simulink model "Sim_PA_DDPG_4drone"  (R2025a)
settings: Solver=ode1  StartTime=0.0  StopTime=Tf  FixedStep=Ts_Sim  RelTol=1e-3
undefined symbols (not defined in the file): control_noise, p_IC, phi_IC, phi_limit, pqr_Limit, psi_dsr, psi_IC, psi_limit, q_IC, r_IC, saturation_logic, state_noise, theta_IC, theta_limit, Ts_Sim, u_IC, uvw_Limit, v_IC, w_IC, wind_logic, x_IC, xy_Limit, y_IC, z_IC, z_Limit
libraries: rllib x8
(part 2 of 2)

== matlab function Sim_PA_DDPG_4drone/leader 1/System Solver/System Solver ==
  data: roll output; pitch output; r_yaw output; ft output; u1 input; u2 input; u3 input; Ts input; r_yaw input
function [roll, pitch, r_yaw, ft ] = system_solver(u1, u2, u3, Ts, r_yaw)

    m = 1; g = 9.81;
    
    ft = m * sqrt( u1^2 + u2^2 + (u3-g)^2 );

    % a = sin(r_yaw);
    % b = cos(r_yaw);
    % 
    % A = u1 / (u3);
    % B = u2 / (u3);
    % C = (a*A - b*B) / ( (a^2) + (b^2)) ;
    % 
    % roll = atan( (B + b*C) / a );
    % pitch = atan( C * cos(roll) );

    roll = asin( (u2*m) / ft );
    pitch = asin( (-u1*m) / (ft*cos(roll)) );
    r_yaw = 0;

    % Smoothing Factor ( Use exponential decay, just to start from zero )
    % roll = roll * (1-exp(-Ts));
    % pitch = pitch * (1-exp(-Ts));
    % r_yaw = r_yaw * (1-exp(-Ts));

    % Saturation
    if roll > pi/10
        roll = pi/10;
    elseif roll < -pi/10
        roll = -pi/10;
    end

    if pitch > pi/10
        pitch = pi/10;
    elseif pitch < -pi/10
        pitch = -pi/10;
    end

end

% function [ft, pitch, roll] = system_solve(u1, u2, u3, psi, m) % u1 = ux , u2 = uy , u3 = uz - g  
%     if psi <= 0.001 && psi >= -0.001
%         psi = 0.001;
%     end
%     a = sin(psi);
%     b = cos(psi);
% 
%     A = u1 / (u3);
%     B = u2 / (u3);
%     C = (a*A - b*B) / ( (a^2) + (b^2)) ;
% 
%     roll = atan( (B + b*C) / a );
%     pitch = atan( C * cos(roll) );
% 
%     % saftey limit threshold on desired pitch and roll
%     if pitch>pi/4
%         pitch = pi/4;
%     elseif pitch<-pi/4
%         pitch = -pi/4;
%     end
%     if roll>pi/4
%         roll = pi/4;
%     elseif roll<-pi/4
%         roll = -pi/4;
%     end
%     ft = ( m / (cos(pitch)*cos(roll)) ) * (-u3); 
% end

== matlab function Sim_PA_DDPG_4drone/leader 1/Attitude DDPG/Attitude Error ==
  data: phi_dsr input; phi_dot_dsr input; theta_dsr input; theta_dot_dsr input; psi_dsr input; psi_dot_dsr input; phi input; theta input; psi input; e_phi output; e_theta output; e_psi output; phi_dot input; theta_dot input; psi_dot input; e_phi_dot output; e_theta_dot output; e_psi_dot output
function [ e_phi, e_theta, e_psi, e_phi_dot, e_theta_dot, e_psi_dot ] = calculate_errors(phi_dsr, phi_dot_dsr, theta_dsr, theta_dot_dsr, psi_dsr, psi_dot_dsr, phi, theta, psi, phi_dot, theta_dot, psi_dot)
   
    e_phi = phi_dsr - phi;
    e_theta = theta_dsr - theta;
    e_psi = psi_dsr - psi;

    e_phi_dot = phi_dot_dsr - phi_dot;
    e_theta_dot = theta_dot_dsr - theta_dot;
    e_psi_dot = psi_dot_dsr - psi_dot;

end

== matlab function Sim_PA_DDPG_4drone/leader 1/Position DDPG/Position Error ==
  data: x_desired input; y_desired input; z_desired input; xdot_desired input; ydot_desired input; zdot_desired input; x input; y input; z input; e_x output; e_y output; e_z output; xdot input; ydot input; zdot input; e_xdot output; e_ydot output; e_zdot output
function [e_x, e_y, e_z, e_xdot, e_ydot, e_zdot] = ...
      calculate_errors(x_desired, y_desired, z_desired, ...
      xdot_desired, ydot_desired, zdot_desired, ...
      x,y,z, xdot,ydot,zdot)

    e_x    = x_desired - x;
    e_y    = y_desired - y;
    e_z    = z_desired - z;
    e_xdot = xdot_desired - xdot;
    e_ydot = ydot_desired - ydot;
    e_zdot = zdot_desired - zdot;
    
end

% formal is Actual - Reference

== matlab function Sim_PA_DDPG_4drone/leader 1/Position DDPG/MATLAB Function ==
  data: e_x input; r output; e_y input; e_z input; e_u input; e_v input; e_w input; u_dot input; v_dot input; w_dot input; isdone output
function [r,isdone] = calculate_reward(e_x, e_y, e_z, e_u, e_v, e_w, u_dot, v_dot, w_dot)

    r = -    1*( abs(e_x)   + abs(e_y)   + abs(e_z) ) ...
        -  0.1*( abs(e_u)   + abs(e_v)   + abs(e_w) ) ...
        - 0.01*( abs(u_dot) + abs(v_dot) + abs(w_dot) );
    
   isdone = 0;
   
end

== matlab function Sim_PA_DDPG_4drone/leader 1/Attitude DDPG/MATLAB Function ==
  data: e_phi input; r output; e_theta input; e_psi input; e_phi_dot input; e_theta_dot input; e_psi_dot input; tau_x input; tau_y input; tau_z input; isdone output
function [r,isdone] = calculate_reward(e_phi, e_theta, e_psi, e_phi_dot, e_theta_dot, e_psi_dot, tau_x, tau_y, tau_z )

    Error_Angle      =    2*( abs(e_phi)     +  abs(e_theta)     + abs(e_psi) );
    Error_Angle_Rate =  0.1*( abs(e_phi_dot) +  abs(e_theta_dot) + abs(e_psi_dot) );
    Action           = 0.01*( abs(tau_x)     +  abs(tau_y)       + abs(tau_z) );

    r = - Error_Angle - Error_Angle_Rate - Action;

    isdone = (abs(e_phi) > 100) || (abs(e_theta) > 100) || (abs(e_psi) > 100);
end

== matlab function Sim_PA_DDPG_4drone/drone 2/Attitude DDPG/MATLAB Function ==
  data: e_phi input; r output; e_theta input; e_psi input; e_phi_dot input; e_theta_dot input; e_psi_dot input; tau_x input; tau_y input; tau_z input; isdone output
function [r,isdone] = calculate_reward(e_phi, e_theta, e_psi, e_phi_dot, e_theta_dot, e_psi_dot, tau_x, tau_y, tau_z )

    Error_Angle      =    2*( abs(e_phi)     +  abs(e_theta)     + abs(e_psi) );
    Error_Angle_Rate =  0.1*( abs(e_phi_dot) +  abs(e_theta_dot) + abs(e_psi_dot) );
    Action           = 0.01*( abs(tau_x)     +  abs(tau_y)       + abs(tau_z) );

    r = - Error_Angle - Error_Angle_Rate - Action;

    isdone = (abs(e_phi) > 100) || (abs(e_theta) > 100) || (abs(e_psi) > 100);
end

== matlab function Sim_PA_DDPG_4drone/drone 2/Drone Dynamics/MATLAB Function ==
  data: ft input; u_dot output; phi input; theta input; psi input; v_dot output; w_dot output
function [u_dot, v_dot, w_dot] = fcn(ft,phi,theta,psi)

m = 1; g = 9.81;

u_dot = -(ft/m)*( sin(phi)*sin(psi) + cos(phi)*cos(psi)*sin(theta) ); 
v_dot = -(ft/m)*( cos(phi)*sin(psi)*sin(theta) - cos(psi)*sin(phi));
w_dot = g-(ft/m)*( cos(phi)*cos(theta) );

end

== matlab function Sim_PA_DDPG_4drone/drone 2/Drone Dynamics/MATLAB Function1 ==
  data: tau_x input; p_dot output; tau_y input; tau_z input; p input; q_dot output; r_dot output; q input; r input
function [p_dot, q_dot, r_dot] = fcn(tau_x,tau_y,tau_z,p,q,r)

Ix = 0.3; Iy = 0.4; Iz = 0.5; 

p_dot = ((Iy-Iz)*q*r/Ix)  + tau_x/Ix;
q_dot = ((Iz-Ix)*p*r/Iy)  + tau_y/Iy;
r_dot = ((Ix-Iy)*p*q/Iz)  + tau_z/Iz;


end

== matlab function Sim_PA_DDPG_4drone/drone 2/Drone Dynamics/MATLAB Function2 ==
  data: p input; q input; r input; phi_dot output; phi input; theta input; theta_dot output; psi_dot output
function [phi_dot, theta_dot, psi_dot] = fcn(p,q,r, phi,theta)

    phi_dot   = p + (q*sin(phi)*tan(theta)) + (r*cos(phi)*tan(theta));
    theta_dot = (q*cos(phi)) - (r*sin(phi));
    psi_dot   = (q*sin(phi)/cos(theta)) + (r*cos(phi)/cos(theta));

end



    % if theta == deg2rad(90) || theta == deg2rad(-90)
    %    theta = sign(theta)*deg2rad(89.9); 
    % end

% 89.9 value is fixed. 
% if change to 89.99, phi_dot and psi_dot value will explode.

== matlab function Sim_PA_DDPG_4drone/drone 2/Drone Dynamics/MATLAB Function3 ==
  settings: updateMethod=DISCRETE
  data: state_vector input; noisy_vector output; noise_percent input
function noisy_vector = add_state_noise(state_vector,noise_percent)

    sensor_uncert = [0.02, 0.02, 0.05, 0.05, 0.05, 0.05, 0.15, 0.15, 0.5, 0.005, 0.005, 0.005]';
  
    noise = (noise_percent) * sensor_uncert .* randn(size(state_vector)); % 0.01 usually add noise_percent 1 2 3 4 5
    noisy_vector = state_vector + noise;

end

== matlab function Sim_PA_DDPG_4drone/drone 2/Drone Dynamics/MATLAB Function4 ==
  settings: updateMethod=DISCRETE
  data: control_vector input; noisy_vector output; noise_percent input
function noisy_vector = add_control_noise(control_vector, noise_percent)

    L = 0.2;
    % drag = 0.02; % (drag coef)
    max_Ft = 2*9.81;
    Tmax = max_Ft/4;
    Max_torque = Tmax*L*2;
    actuator_uncert = [0.1*max_Ft, 0.01*Max_torque, 0.01*Max_torque, 0.02*Max_torque]';
    
    noise = (noise_percent) * actuator_uncert .* randn(size(control_vector)); % noise_percent 1 2 3 4 5
    noisy_vector = control_vector + noise;
    
end

== matlab function Sim_PA_DDPG_4drone/drone 2/Drone Dynamics/MATLAB Function5 ==
  data: X input; Wxyz input; X output; Ts_Sim input; wind_logic input
function X = wind_f_m( X,Wxyz, Ts_Sim,  wind_logic)

    Cd = [.8; 0.8;1.2]; % Drag coefficient
    L = 0.2; % Half arm length (m)
    h = 0.05;
    A = [L*2*h, L*2*h, 2*L*L]; % Approximate frontal areas [x, y, z] in m^2
    r = [ L,  L, -L, -L;   % X positions of motors
          L, -L, -L,  L;   % Y positions of motors
          0,  0,  0,  0 ]; % Z positions (motors at same height)
    rho = 1.225; % Air density (kg/m^3)

    Ix = 0.3; Iy = 0.4; Iz = 0.5; m = 1;
    if wind_logic ==1
        R = eul2rotm_zyx( X(7), X(8), X(9) );
        Wxyz_body = R'*Wxyz;
        V_rel = X(4:6) - Wxyz_body;
        F_wind = -0.5 * rho * Cd .*diag(A) * (V_rel .* abs(V_rel)); % Compute wind forces
        
        F_wind_motors = repmat(F_wind, 1, 4) + 0.01*randn(3,4);
    
        M_wind_motors = cross(r, F_wind_motors, 1);
        M_wind = sum(M_wind_motors, 2);  
        
        accn_dist = F_wind/m;
        alpha_dist=    [M_wind(1)/Ix;
                        M_wind(2)/Iy;
                        M_wind(3)/Iz];
    
        X = X + Ts_Sim * [0;0;0;
                         accn_dist;
                         0;0;0;
                         alpha_dist];
    end
end

== matlab function Sim_PA_DDPG_4drone/drone 2/Drone Dynamics/MATLAB Function6 ==
  data: U input; out output; logic input
% saturation function
function out = saturate_controls(U, logic)

    if logic == 1

        ft = U(1);
        torques = [U(2); U(3); U(4)];
        m = 1;
        g = 9.81;
        L = 0.2;
        drag = 0.02; % (drag coef)
        max_Ft = 2*m*g;
        Tmin = 0;
        Tmax = max_Ft/4;
        max_torque = Tmax*L*2;
        max_yaw_torque = 0.7*max_torque;

        % saturate the torques to the max torque the drone can produce
        for p = 1:2 % sat the first 2
            if torques(p) > max_torque
                torques(p) = max_torque;
            elseif torques(p) < -max_torque
                torques(p) = -max_torque;
            end
        end
        if torques(3) > max_yaw_torque
            torques(3) = max_yaw_torque;
        elseif torques(3) < -max_yaw_torque
            torques(3) = -max_yaw_torque;
        end
        % solve for the thrust of each motor given those torques
        T1 = (ft - torques(1)/(2*L) - torques(2)/(2*L) + torques(3)/(4*drag)) / 4;
        T2 = (ft - torques(1)/(2*L) + torques(2)/(2*L) + torques(3)/(4*drag)) / 4;
        T3 = (ft + torques(1)/(2*L) - torques(2)/(2*L) - torques(3)/(4*drag)) / 4;
        T4 = (ft + torques(1)/(2*L) + torques(2)/(2*L) - torques(3)/(4*drag)) / 4;
        each_motor_thrust = [T1;T2;T3;T4];

        % saturate each motor thrust to its bounded values
        for j = 1:4
            if each_motor_thrust(j) > Tmax
                each_motor_thrust(j) = Tmax;
            elseif each_motor_thrust(j) < Tmin
                each_motor_thrust(j) = Tmin;
            end
        end

        ft = sum(each_motor_thrust);

        if ft>max_Ft
            ft = max_Ft;
        elseif ft<0
            ft = 0;
        end

        out = [ft; torques];

    else
    
        out = U;
    
    end


end

== matlab function Sim_PA_DDPG_4drone/drone 2/Position DDPG/MATLAB Function ==
  data: e_x input; r output; e_y input; e_z input; e_u input; e_v input; e_w input; u_dot input; v_dot input; w_dot input; isdone output
function [r,isdone] = calculate_reward(e_x, e_y, e_z, e_u, e_v, e_w, u_dot, v_dot, w_dot)

    r = -    1*( abs(e_x)   + abs(e_y)   + abs(e_z) ) ...
        -  0.1*( abs(e_u)   + abs(e_v)   + abs(e_w) ) ...
        - 0.01*( abs(u_dot) + abs(v_dot) + abs(w_dot) );
    
   isdone = 0;
   
end

== matlab function Sim_PA_DDPG_4drone/leader 1/Drone Dynamics/MATLAB Function1 ==
  data: tau_x input; p_dot output; tau_y input; tau_z input; p input; q_dot output; r_dot output; q input; r input
function [p_dot, q_dot, r_dot] = fcn(tau_x,tau_y,tau_z,p,q,r)

Ix = 0.3; Iy = 0.4; Iz = 0.5; 

p_dot = ((Iy-Iz)*q*r/Ix)  + tau_x/Ix;
q_dot = ((Iz-Ix)*p*r/Iy)  + tau_y/Iy;
r_dot = ((Ix-Iy)*p*q/Iz)  + tau_z/Iz;


end

== matlab function Sim_PA_DDPG_4drone/drone 2/Position DDPG/Position Error ==
  data: x_desired input; y_desired input; z_desired input; xdot_desired input; ydot_desired input; zdot_desired input; x input; y input; z input; e_x output; e_y output; e_z output; xdot input; ydot input; zdot input; e_xdot output; e_ydot output; e_zdot output
function [e_x, e_y, e_z, e_xdot, e_ydot, e_zdot] = ...
      calculate_errors(x_desired, y_desired, z_desired, ...
      xdot_desired, ydot_desired, zdot_desired, ...
      x,y,z, xdot,ydot,zdot)

    e_x    = x_desired - x;
    e_y    = y_desired - y;
    e_z    = z_desired - z;
    e_xdot = xdot_desired - xdot;
    e_ydot = ydot_desired - ydot;
    e_zdot = zdot_desired - zdot;
    
end

% formal is Actual - Reference

== matlab function Sim_PA_DDPG_4drone/drone 2/System Solver/System Solver ==
  data: roll output; pitch output; r_yaw output; ft output; u1 input; u2 input; u3 input; Ts input; r_yaw input
function [roll, pitch, r_yaw, ft ] = system_solver(u1, u2, u3, Ts, r_yaw)

    m = 1; g = 9.81;
    
    ft = m * sqrt( u1^2 + u2^2 + (u3-g)^2 );

    % a = sin(r_yaw);
    % b = cos(r_yaw);
    % 
    % A = u1 / (u3);
    % B = u2 / (u3);
    % C = (a*A - b*B) / ( (a^2) + (b^2)) ;
    % 
    % roll = atan( (B + b*C) / a );
    % pitch = atan( C * cos(roll) );

    roll = asin( (u2*m) / ft );
    pitch = asin( (-u1*m) / (ft*cos(roll)) );
    r_yaw = 0;

    % Smoothing Factor ( Use exponential decay, just to start from zero )
    % roll = roll * (1-exp(-Ts));
    % pitch = pitch * (1-exp(-Ts));
    % r_yaw = r_yaw * (1-exp(-Ts));

    % Saturation
    if roll > pi/10
        roll = pi/10;
    elseif roll < -pi/10
        roll = -pi/10;
    end

    if pitch > pi/10
        pitch = pi/10;
    elseif pitch < -pi/10
        pitch = -pi/10;
    end

end

% function [ft, pitch, roll] = system_solve(u1, u2, u3, psi, m) % u1 = ux , u2 = uy , u3 = uz - g  
%     if psi <= 0.001 && psi >= -0.001
%         psi = 0.001;
%     end
%     a = sin(psi);
%     b = cos(psi);
% 
%     A = u1 / (u3);
%     B = u2 / (u3);
%     C = (a*A - b*B) / ( (a^2) + (b^2)) ;
% 
%     roll = atan( (B + b*C) / a );
%     pitch = atan( C * cos(roll) );
% 
%     % saftey limit threshold on desired pitch and roll
%     if pitch>pi/4
%         pitch = pi/4;
%     elseif pitch<-pi/4
%         pitch = -pi/4;
%     end
%     if roll>pi/4
%         roll = pi/4;
%     elseif roll<-pi/4
%         roll = -pi/4;
%     end
%     ft = ( m / (cos(pitch)*cos(roll)) ) * (-u3); 
% end

== matlab function Sim_PA_DDPG_4drone/drone 3/Attitude DDPG/Attitude Error ==
  data: phi_dsr input; phi_dot_dsr input; theta_dsr input; theta_dot_dsr input; psi_dsr input; psi_dot_dsr input; phi input; theta input; psi input; e_phi output; e_theta output; e_psi output; phi_dot input; theta_dot input; psi_dot input; e_phi_dot output; e_theta_dot output; e_psi_dot output
function [ e_phi, e_theta, e_psi, e_phi_dot, e_theta_dot, e_psi_dot ] = calculate_errors(phi_dsr, phi_dot_dsr, theta_dsr, theta_dot_dsr, psi_dsr, psi_dot_dsr, phi, theta, psi, phi_dot, theta_dot, psi_dot)
   
    e_phi = phi_dsr - phi;
    e_theta = theta_dsr - theta;
    e_psi = psi_dsr - psi;

    e_phi_dot = phi_dot_dsr - phi_dot;
    e_theta_dot = theta_dot_dsr - theta_dot;
    e_psi_dot = psi_dot_dsr - psi_dot;

end

== matlab function Sim_PA_DDPG_4drone/drone 3/Attitude DDPG/MATLAB Function ==
  data: e_phi input; r output; e_theta input; e_psi input; e_phi_dot input; e_theta_dot input; e_psi_dot input; tau_x input; tau_y input; tau_z input; isdone output
function [r,isdone] = calculate_reward(e_phi, e_theta, e_psi, e_phi_dot, e_theta_dot, e_psi_dot, tau_x, tau_y, tau_z )

    Error_Angle      =    2*( abs(e_phi)     +  abs(e_theta)     + abs(e_psi) );
    Error_Angle_Rate =  0.1*( abs(e_phi_dot) +  abs(e_theta_dot) + abs(e_psi_dot) );
    Action           = 0.01*( abs(tau_x)     +  abs(tau_y)       + abs(tau_z) );

    r = - Error_Angle - Error_Angle_Rate - Action;

    isdone = (abs(e_phi) > 100) || (abs(e_theta) > 100) || (abs(e_psi) > 100);
end

== matlab function Sim_PA_DDPG_4drone/drone 3/Drone Dynamics/MATLAB Function ==
  data: ft input; u_dot output; phi input; theta input; psi input; v_dot output; w_dot output
function [u_dot, v_dot, w_dot] = fcn(ft,phi,theta,psi)

m = 1; g = 9.81;

u_dot = -(ft/m)*( sin(phi)*sin(psi) + cos(phi)*cos(psi)*sin(theta) ); 
v_dot = -(ft/m)*( cos(phi)*sin(psi)*sin(theta) - cos(psi)*sin(phi));
w_dot = g-(ft/m)*( cos(phi)*cos(theta) );

end

== matlab function Sim_PA_DDPG_4drone/drone 3/Drone Dynamics/MATLAB Function1 ==
  data: tau_x input; p_dot output; tau_y input; tau_z input; p input; q_dot output; r_dot output; q input; r input
function [p_dot, q_dot, r_dot] = fcn(tau_x,tau_y,tau_z,p,q,r)

Ix = 0.3; Iy = 0.4; Iz = 0.5; 

p_dot = ((Iy-Iz)*q*r/Ix)  + tau_x/Ix;
q_dot = ((Iz-Ix)*p*r/Iy)  + tau_y/Iy;
r_dot = ((Ix-Iy)*p*q/Iz)  + tau_z/Iz;


end

== matlab function Sim_PA_DDPG_4drone/drone 3/Drone Dynamics/MATLAB Function2 ==
  data: p input; q input; r input; phi_dot output; phi input; theta input; theta_dot output; psi_dot output
function [phi_dot, theta_dot, psi_dot] = fcn(p,q,r, phi,theta)

    phi_dot   = p + (q*sin(phi)*tan(theta)) + (r*cos(phi)*tan(theta));
    theta_dot = (q*cos(phi)) - (r*sin(phi));
    psi_dot   = (q*sin(phi)/cos(theta)) + (r*cos(phi)/cos(theta));

end



    % if theta == deg2rad(90) || theta == deg2rad(-90)
    %    theta = sign(theta)*deg2rad(89.9); 
    % end

% 89.9 value is fixed. 
% if change to 89.99, phi_dot and psi_dot value will explode.

== matlab function Sim_PA_DDPG_4drone/drone 3/Drone Dynamics/MATLAB Function3 ==
  settings: updateMethod=DISCRETE
  data: state_vector input; noisy_vector output; noise_percent input
function noisy_vector = add_state_noise(state_vector,noise_percent)

    sensor_uncert = [0.02, 0.02, 0.05, 0.05, 0.05, 0.05, 0.15, 0.15, 0.5, 0.005, 0.005, 0.005]';
  
    noise = (noise_percent) * sensor_uncert .* randn(size(state_vector)); % 0.01 usually add noise_percent 1 2 3 4 5
    noisy_vector = state_vector + noise;

end

== matlab function Sim_PA_DDPG_4drone/drone 3/Drone Dynamics/MATLAB Function4 ==
  settings: updateMethod=DISCRETE
  data: control_vector input; noisy_vector output; noise_percent input
function noisy_vector = add_control_noise(control_vector, noise_percent)

    L = 0.2;
    % drag = 0.02; % (drag coef)
    max_Ft = 2*9.81;
    Tmax = max_Ft/4;
    Max_torque = Tmax*L*2;
    actuator_uncert = [0.1*max_Ft, 0.01*Max_torque, 0.01*Max_torque, 0.02*Max_torque]';
    
    noise = (noise_percent) * actuator_uncert .* randn(size(control_vector)); % noise_percent 1 2 3 4 5
    noisy_vector = control_vector + noise;
    
end

== matlab function Sim_PA_DDPG_4drone/leader 1/Drone Dynamics/MATLAB Function ==
  data: ft input; u_dot output; phi input; theta input; psi input; v_dot output; w_dot output
function [u_dot, v_dot, w_dot] = fcn(ft,phi,theta,psi)

m = 1; g = 9.81;

u_dot = -(ft/m)*( sin(phi)*sin(psi) + cos(phi)*cos(psi)*sin(theta) ); 
v_dot = -(ft/m)*( cos(phi)*sin(psi)*sin(theta) - cos(psi)*sin(phi));
w_dot = g-(ft/m)*( cos(phi)*cos(theta) );

end

== matlab function Sim_PA_DDPG_4drone/drone 3/Drone Dynamics/MATLAB Function5 ==
  data: X input; Wxyz input; X output; Ts_Sim input; wind_logic input
function X = wind_f_m( X,Wxyz, Ts_Sim,  wind_logic)

    Cd = [.8; 0.8;1.2]; % Drag coefficient
    L = 0.2; % Half arm length (m)
    h = 0.05;
    A = [L*2*h, L*2*h, 2*L*L]; % Approximate frontal areas [x, y, z] in m^2
    r = [ L,  L, -L, -L;   % X positions of motors
          L, -L, -L,  L;   % Y positions of motors
          0,  0,  0,  0 ]; % Z positions (motors at same height)
    rho = 1.225; % Air density (kg/m^3)

    Ix = 0.3; Iy = 0.4; Iz = 0.5; m = 1;
    if wind_logic ==1
        R = eul2rotm_zyx( X(7), X(8), X(9) );
        Wxyz_body = R'*Wxyz;
        V_rel = X(4:6) - Wxyz_body;
        F_wind = -0.5 * rho * Cd .*diag(A) * (V_rel .* abs(V_rel)); % Compute wind forces
        
        F_wind_motors = repmat(F_wind, 1, 4) + 0.01*randn(3,4);
    
        M_wind_motors = cross(r, F_wind_motors, 1);
        M_wind = sum(M_wind_motors, 2);  
        
        accn_dist = F_wind/m;
        alpha_dist=    [M_wind(1)/Ix;
                        M_wind(2)/Iy;
                        M_wind(3)/Iz];
    
        X = X + Ts_Sim * [0;0;0;
                         accn_dist;
                         0;0;0;
                         alpha_dist];
    end
end

== matlab function Sim_PA_DDPG_4drone/drone 3/Drone Dynamics/MATLAB Function6 ==
  data: U input; out output; logic input
% saturation function
function out = saturate_controls(U, logic)

    if logic == 1

        ft = U(1);
        torques = [U(2); U(3); U(4)];
        m = 1;
        g = 9.81;
        L = 0.2;
        drag = 0.02; % (drag coef)
        max_Ft = 2*m*g;
        Tmin = 0;
        Tmax = max_Ft/4;
        max_torque = Tmax*L*2;
        max_yaw_torque = 0.7*max_torque;

        % saturate the torques to the max torque the drone can produce
        for p = 1:2 % sat the first 2
            if torques(p) > max_torque
                torques(p) = max_torque;
            elseif torques(p) < -max_torque
                torques(p) = -max_torque;
            end
        end
        if torques(3) > max_yaw_torque
            torques(3) = max_yaw_torque;
        elseif torques(3) < -max_yaw_torque
            torques(3) = -max_yaw_torque;
        end
        % solve for the thrust of each motor given those torques
        T1 = (ft - torques(1)/(2*L) - torques(2)/(2*L) + torques(3)/(4*drag)) / 4;
        T2 = (ft - torques(1)/(2*L) + torques(2)/(2*L) + torques(3)/(4*drag)) / 4;
        T3 = (ft + torques(1)/(2*L) - torques(2)/(2*L) - torques(3)/(4*drag)) / 4;
        T4 = (ft + torques(1)/(2*L) + torques(2)/(2*L) - torques(3)/(4*drag)) / 4;
        each_motor_thrust = [T1;T2;T3;T4];

        % saturate each motor thrust to its bounded values
        for j = 1:4
            if each_motor_thrust(j) > Tmax
                each_motor_thrust(j) = Tmax;
            elseif each_motor_thrust(j) < Tmin
                each_motor_thrust(j) = Tmin;
            end
        end

        ft = sum(each_motor_thrust);

        if ft>max_Ft
            ft = max_Ft;
        elseif ft<0
            ft = 0;
        end

        out = [ft; torques];

    else
    
        out = U;
    
    end


end

== matlab function Sim_PA_DDPG_4drone/drone 3/Position DDPG/MATLAB Function ==
  data: e_x input; r output; e_y input; e_z input; e_u input; e_v input; e_w input; u_dot input; v_dot input; w_dot input; isdone output
function [r,isdone] = calculate_reward(e_x, e_y, e_z, e_u, e_v, e_w, u_dot, v_dot, w_dot)

    r = -    1*( abs(e_x)   + abs(e_y)   + abs(e_z) ) ...
        -  0.1*( abs(e_u)   + abs(e_v)   + abs(e_w) ) ...
        - 0.01*( abs(u_dot) + abs(v_dot) + abs(w_dot) );
    
   isdone = 0;
   
end

== matlab function Sim_PA_DDPG_4drone/drone 3/Position DDPG/Position Error ==
  data: x_desired input; y_desired input; z_desired input; xdot_desired input; ydot_desired input; zdot_desired input; x input; y input; z input; e_x output; e_y output; e_z output; xdot input; ydot input; zdot input; e_xdot output; e_ydot output; e_zdot output
function [e_x, e_y, e_z, e_xdot, e_ydot, e_zdot] = ...
      calculate_errors(x_desired, y_desired, z_desired, ...
      xdot_desired, ydot_desired, zdot_desired, ...
      x,y,z, xdot,ydot,zdot)

    e_x    = x_desired - x;
    e_y    = y_desired - y;
    e_z    = z_desired - z;
    e_xdot = xdot_desired - xdot;
    e_ydot = ydot_desired - ydot;
    e_zdot = zdot_desired - zdot;
    
end

% formal is Actual - Reference

== matlab function Sim_PA_DDPG_4drone/drone 3/System Solver/System Solver ==
  data: roll output; pitch output; r_yaw output; ft output; u1 input; u2 input; u3 input; Ts input; r_yaw input
function [roll, pitch, r_yaw, ft ] = system_solver(u1, u2, u3, Ts, r_yaw)

    m = 1; g = 9.81;
    
    ft = m * sqrt( u1^2 + u2^2 + (u3-g)^2 );

    % a = sin(r_yaw);
    % b = cos(r_yaw);
    % 
    % A = u1 / (u3);
    % B = u2 / (u3);
    % C = (a*A - b*B) / ( (a^2) + (b^2)) ;
    % 
    % roll = atan( (B + b*C) / a );
    % pitch = atan( C * cos(roll) );

    roll = asin( (u2*m) / ft );
    pitch = asin( (-u1*m) / (ft*cos(roll)) );
    r_yaw = 0;

    % Smoothing Factor ( Use exponential decay, just to start from zero )
    % roll = roll * (1-exp(-Ts));
    % pitch = pitch * (1-exp(-Ts));
    % r_yaw = r_yaw * (1-exp(-Ts));

    % Saturation
    if roll > pi/10
        roll = pi/10;
    elseif roll < -pi/10
        roll = -pi/10;
    end

    if pitch > pi/10
        pitch = pi/10;
    elseif pitch < -pi/10
        pitch = -pi/10;
    end

end

% function [ft, pitch, roll] = system_solve(u1, u2, u3, psi, m) % u1 = ux , u2 = uy , u3 = uz - g  
%     if psi <= 0.001 && psi >= -0.001
%         psi = 0.001;
%     end
%     a = sin(psi);
%     b = cos(psi);
% 
%     A = u1 / (u3);
%     B = u2 / (u3);
%     C = (a*A - b*B) / ( (a^2) + (b^2)) ;
% 
%     roll = atan( (B + b*C) / a );
%     pitch = atan( C * cos(roll) );
% 
%     % saftey limit threshold on desired pitch and roll
%     if pitch>pi/4
%         pitch = pi/4;
%     elseif pitch<-pi/4
%         pitch = -pi/4;
%     end
%     if roll>pi/4
%         roll = pi/4;
%     elseif roll<-pi/4
%         roll = -pi/4;
%     end
%     ft = ( m / (cos(pitch)*cos(roll)) ) * (-u3); 
% end

== matlab function Sim_PA_DDPG_4drone/drone 4/Attitude DDPG/Attitude Error ==
  data: phi_dsr input; phi_dot_dsr input; theta_dsr input; theta_dot_dsr input; psi_dsr input; psi_dot_dsr input; phi input; theta input; psi input; e_phi output; e_theta output; e_psi output; phi_dot input; theta_dot input; psi_dot input; e_phi_dot output; e_theta_dot output; e_psi_dot output
function [ e_phi, e_theta, e_psi, e_phi_dot, e_theta_dot, e_psi_dot ] = calculate_errors(phi_dsr, phi_dot_dsr, theta_dsr, theta_dot_dsr, psi_dsr, psi_dot_dsr, phi, theta, psi, phi_dot, theta_dot, psi_dot)
   
    e_phi = phi_dsr - phi;
    e_theta = theta_dsr - theta;
    e_psi = psi_dsr - psi;

    e_phi_dot = phi_dot_dsr - phi_dot;
    e_theta_dot = theta_dot_dsr - theta_dot;
    e_psi_dot = psi_dot_dsr - psi_dot;

end

== matlab function Sim_PA_DDPG_4drone/drone 4/Attitude DDPG/MATLAB Function ==
  data: e_phi input; r output; e_theta input; e_psi input; e_phi_dot input; e_theta_dot input; e_psi_dot input; tau_x input; tau_y input; tau_z input; isdone output
function [r,isdone] = calculate_reward(e_phi, e_theta, e_psi, e_phi_dot, e_theta_dot, e_psi_dot, tau_x, tau_y, tau_z )

    Error_Angle      =    2*( abs(e_phi)     +  abs(e_theta)     + abs(e_psi) );
    Error_Angle_Rate =  0.1*( abs(e_phi_dot) +  abs(e_theta_dot) + abs(e_psi_dot) );
    Action           = 0.01*( abs(tau_x)     +  abs(tau_y)       + abs(tau_z) );

    r = - Error_Angle - Error_Angle_Rate - Action;

    isdone = (abs(e_phi) > 100) || (abs(e_theta) > 100) || (abs(e_psi) > 100);
end

== matlab function Sim_PA_DDPG_4drone/drone 4/Drone Dynamics/MATLAB Function ==
  data: ft input; u_dot output; phi input; theta input; psi input; v_dot output; w_dot output
function [u_dot, v_dot, w_dot] = fcn(ft,phi,theta,psi)

m = 1; g = 9.81;

u_dot = -(ft/m)*( sin(phi)*sin(psi) + cos(phi)*cos(psi)*sin(theta) ); 
v_dot = -(ft/m)*( cos(phi)*sin(psi)*sin(theta) - cos(psi)*sin(phi));
w_dot = g-(ft/m)*( cos(phi)*cos(theta) );

end

== matlab function Sim_PA_DDPG_4drone/leader 1/Drone Dynamics/MATLAB Function2 ==
  data: p input; q input; r input; phi_dot output; phi input; theta input; theta_dot output; psi_dot output
function [phi_dot, theta_dot, psi_dot] = fcn(p,q,r, phi,theta)

    phi_dot   = p + (q*sin(phi)*tan(theta)) + (r*cos(phi)*tan(theta));
    theta_dot = (q*cos(phi)) - (r*sin(phi));
    psi_dot   = (q*sin(phi)/cos(theta)) + (r*cos(phi)/cos(theta));

end



    % if theta == deg2rad(90) || theta == deg2rad(-90)
    %    theta = sign(theta)*deg2rad(89.9); 
    % end

% 89.9 value is fixed. 
% if change to 89.99, phi_dot and psi_dot value will explode.

== matlab function Sim_PA_DDPG_4drone/drone 4/Drone Dynamics/MATLAB Function1 ==
  data: tau_x input; p_dot output; tau_y input; tau_z input; p input; q_dot output; r_dot output; q input; r input
function [p_dot, q_dot, r_dot] = fcn(tau_x,tau_y,tau_z,p,q,r)

Ix = 0.3; Iy = 0.4; Iz = 0.5; 

p_dot = ((Iy-Iz)*q*r/Ix)  + tau_x/Ix;
q_dot = ((Iz-Ix)*p*r/Iy)  + tau_y/Iy;
r_dot = ((Ix-Iy)*p*q/Iz)  + tau_z/Iz;


end

== matlab function Sim_PA_DDPG_4drone/Ref Mixer ==
  data: t input; leader input; drone2 input; drone3 input; drone4 input; ref2 output; ref3 output; ref4 output
function [ref2, ref3, ref4] = fcn(t, leader, drone2, drone3, drone4)
ref2 = zeros(6,1);
ref3 = zeros(6,1);
ref4 = zeros(6,1);
N = 5000;
N1 = floor(N/3);
N2 = floor(2*N/3);

comm = 1;
offsets = zeros(3, 4);
offsets(:,1) = [ 0;  0; 0];
offsets(:,2) = [-1;  0; 0];
offsets(:,3) = [-1; -1; 0];
offsets(:,4) = [-1;  1; 0];
X1 = zeros(6,1);
X2 = zeros(6,1);
X3 = zeros(6,1);
X4 = zeros(6,1);

X1 = [leader(1); leader(2); leader(3);leader(4);leader(5);leader(6)];
X2 = [drone2(1);drone2(2);drone2(3);drone2(4);drone2(5);drone2(6)];
X3 = [drone3(1);drone3(2);drone3(3);drone3(4);drone3(5);drone3(6)];
X4 = [drone4(1);drone4(2);drone4(3);drone4(4);drone4(5);drone4(6)];

    if comm == 0
        ref2 = [X1(1:3) + offsets(:,2); X1(4:6)];
        ref3 = [X1(1:3) + offsets(:,3); X1(4:6)];
        ref4 = [X1(1:3) + offsets(:,4); X1(4:6)];
    elseif comm == 1
        if t <= (N1/2)*.01
            ref2 = [X1(1:3) + offsets(:,2); X1(4:6)];
            ref3 = [X1(1:3) + offsets(:,3); X1(4:6)];
            ref4 = [X1(1:3) + offsets(:,4); X1(4:6)];
        elseif t <= N1*.01 && t > (N1/2)*.01
            ref2 = [X3(1:3) + (offsets(:,2) - offsets(:,3));   X3(4:6)]; % 2 only sees 3
            ref3 = [X1(1:3) + offsets(:,3);                    X1(4:6)]; % 2 only sees leader
            ref4 = [X2(1:3) + (offsets(:,4) - offsets(:,2));   X2(4:6)]; % 4 only sees 2
        elseif t <= N2*.01 && t > N1*.01
            ref2 = [X1(1:3) + offsets(:,2);                    X1(4:6)]; % 2 only sees leader
            ref3 = [X2(1:3) + (offsets(:,3) - offsets(:,2));   X2(4:6)]; % 3 only sees 2
            ref4 = [X3(1:3) + (offsets(:,4) - offsets(:,3));   X3(4:6)]; % 4 only sees 3
        else
            ref2 = [X3(1:3) + (offsets(:,2) - offsets(:,3));   X3(4:6)]; % 2 only sees 3
            ref3 = [(X4(1:3) + (offsets(:,3)- offsets(:,4)));  X4(4:6)]; % 3 only sees 4
            ref4 = [X1(1:3) + offsets(:,4);                    X1(4:6)]; % 4 only sees leader
        end

    end
end

== matlab function Sim_PA_DDPG_4drone/drone 4/Drone Dynamics/MATLAB Function2 ==
  data: p input; q input; r input; phi_dot output; phi input; theta input; theta_dot output; psi_dot output
function [phi_dot, theta_dot, psi_dot] = fcn(p,q,r, phi,theta)

    phi_dot   = p + (q*sin(phi)*tan(theta)) + (r*cos(phi)*tan(theta));
    theta_dot = (q*cos(phi)) - (r*sin(phi));
    psi_dot   = (q*sin(phi)/cos(theta)) + (r*cos(phi)/cos(theta));

end



    % if theta == deg2rad(90) || theta == deg2rad(-90)
    %    theta = sign(theta)*deg2rad(89.9); 
    % end

% 89.9 value is fixed. 
% if change to 89.99, phi_dot and psi_dot value will explode.

== matlab function Sim_PA_DDPG_4drone/drone 4/Drone Dynamics/MATLAB Function3 ==
  settings: updateMethod=DISCRETE
  data: state_vector input; noisy_vector output; noise_percent input
function noisy_vector = add_state_noise(state_vector,noise_percent)

    sensor_uncert = [0.02, 0.02, 0.05, 0.05, 0.05, 0.05, 0.15, 0.15, 0.5, 0.005, 0.005, 0.005]';
  
    noise = (noise_percent) * sensor_uncert .* randn(size(state_vector)); % 0.01 usually add noise_percent 1 2 3 4 5
    noisy_vector = state_vector + noise;

end

== matlab function Sim_PA_DDPG_4drone/drone 4/Drone Dynamics/MATLAB Function4 ==
  settings: updateMethod=DISCRETE
  data: control_vector input; noisy_vector output; noise_percent input
function noisy_vector = add_control_noise(control_vector, noise_percent)

    L = 0.2;
    % drag = 0.02; % (drag coef)
    max_Ft = 2*9.81;
    Tmax = max_Ft/4;
    Max_torque = Tmax*L*2;
    actuator_uncert = [0.1*max_Ft, 0.01*Max_torque, 0.01*Max_torque, 0.02*Max_torque]';
    
    noise = (noise_percent) * actuator_uncert .* randn(size(control_vector)); % noise_percent 1 2 3 4 5
    noisy_vector = control_vector + noise;
    
end

== matlab function Sim_PA_DDPG_4drone/drone 4/Drone Dynamics/MATLAB Function5 ==
  data: X input; Wxyz input; X output; Ts_Sim input; wind_logic input
function X = wind_f_m( X,Wxyz, Ts_Sim,  wind_logic)

    Cd = [.8; 0.8;1.2]; % Drag coefficient
    L = 0.2; % Half arm length (m)
    h = 0.05;
    A = [L*2*h, L*2*h, 2*L*L]; % Approximate frontal areas [x, y, z] in m^2
    r = [ L,  L, -L, -L;   % X positions of motors
          L, -L, -L,  L;   % Y positions of motors
          0,  0,  0,  0 ]; % Z positions (motors at same height)
    rho = 1.225; % Air density (kg/m^3)

    Ix = 0.3; Iy = 0.4; Iz = 0.5; m = 1;
    if wind_logic ==1
        R = eul2rotm_zyx( X(7), X(8), X(9) );
        Wxyz_body = R'*Wxyz;
        V_rel = X(4:6) - Wxyz_body;
        F_wind = -0.5 * rho * Cd .*diag(A) * (V_rel .* abs(V_rel)); % Compute wind forces
        
        F_wind_motors = repmat(F_wind, 1, 4) + 0.01*randn(3,4);
    
        M_wind_motors = cross(r, F_wind_motors, 1);
        M_wind = sum(M_wind_motors, 2);  
        
        accn_dist = F_wind/m;
        alpha_dist=    [M_wind(1)/Ix;
                        M_wind(2)/Iy;
                        M_wind(3)/Iz];
    
        X = X + Ts_Sim * [0;0;0;
                         accn_dist;
                         0;0;0;
                         alpha_dist];
    end
end

== matlab function Sim_PA_DDPG_4drone/drone 4/Drone Dynamics/MATLAB Function6 ==
  data: U input; out output; logic input
% saturation function
function out = saturate_controls(U, logic)

    if logic == 1

        ft = U(1);
        torques = [U(2); U(3); U(4)];
        m = 1;
        g = 9.81;
        L = 0.2;
        drag = 0.02; % (drag coef)
        max_Ft = 2*m*g;
        Tmin = 0;
        Tmax = max_Ft/4;
        max_torque = Tmax*L*2;
        max_yaw_torque = 0.7*max_torque;

        % saturate the torques to the max torque the drone can produce
        for p = 1:2 % sat the first 2
            if torques(p) > max_torque
                torques(p) = max_torque;
            elseif torques(p) < -max_torque
                torques(p) = -max_torque;
            end
        end
        if torques(3) > max_yaw_torque
            torques(3) = max_yaw_torque;
        elseif torques(3) < -max_yaw_torque
            torques(3) = -max_yaw_torque;
        end
        % solve for the thrust of each motor given those torques
        T1 = (ft - torques(1)/(2*L) - torques(2)/(2*L) + torques(3)/(4*drag)) / 4;
        T2 = (ft - torques(1)/(2*L) + torques(2)/(2*L) + torques(3)/(4*drag)) / 4;
        T3 = (ft + torques(1)/(2*L) - torques(2)/(2*L) - torques(3)/(4*drag)) / 4;
        T4 = (ft + torques(1)/(2*L) + torques(2)/(2*L) - torques(3)/(4*drag)) / 4;
        each_motor_thrust = [T1;T2;T3;T4];

        % saturate each motor thrust to its bounded values
        for j = 1:4
            if each_motor_thrust(j) > Tmax
                each_motor_thrust(j) = Tmax;
            elseif each_motor_thrust(j) < Tmin
                each_motor_thrust(j) = Tmin;
            end
        end

        ft = sum(each_motor_thrust);

        if ft>max_Ft
            ft = max_Ft;
        elseif ft<0
            ft = 0;
        end

        out = [ft; torques];

    else
    
        out = U;
    
    end


end

== matlab function Sim_PA_DDPG_4drone/drone 4/Position DDPG/MATLAB Function ==
  data: e_x input; r output; e_y input; e_z input; e_u input; e_v input; e_w input; u_dot input; v_dot input; w_dot input; isdone output
function [r,isdone] = calculate_reward(e_x, e_y, e_z, e_u, e_v, e_w, u_dot, v_dot, w_dot)

    r = -    1*( abs(e_x)   + abs(e_y)   + abs(e_z) ) ...
        -  0.1*( abs(e_u)   + abs(e_v)   + abs(e_w) ) ...
        - 0.01*( abs(u_dot) + abs(v_dot) + abs(w_dot) );
    
   isdone = 0;
   
end

== matlab function Sim_PA_DDPG_4drone/drone 4/Position DDPG/Position Error ==
  data: x_desired input; y_desired input; z_desired input; xdot_desired input; ydot_desired input; zdot_desired input; x input; y input; z input; e_x output; e_y output; e_z output; xdot input; ydot input; zdot input; e_xdot output; e_ydot output; e_zdot output
function [e_x, e_y, e_z, e_xdot, e_ydot, e_zdot] = ...
      calculate_errors(x_desired, y_desired, z_desired, ...
      xdot_desired, ydot_desired, zdot_desired, ...
      x,y,z, xdot,ydot,zdot)

    e_x    = x_desired - x;
    e_y    = y_desired - y;
    e_z    = z_desired - z;
    e_xdot = xdot_desired - xdot;
    e_ydot = ydot_desired - ydot;
    e_zdot = zdot_desired - zdot;
    
end

% formal is Actual - Reference

== matlab function Sim_PA_DDPG_4drone/drone 4/System Solver/System Solver ==
  data: roll output; pitch output; r_yaw output; ft output; u1 input; u2 input; u3 input; Ts input; r_yaw input
function [roll, pitch, r_yaw, ft ] = system_solver(u1, u2, u3, Ts, r_yaw)

    m = 1; g = 9.81;
    
    ft = m * sqrt( u1^2 + u2^2 + (u3-g)^2 );

    % a = sin(r_yaw);
    % b = cos(r_yaw);
    % 
    % A = u1 / (u3);
    % B = u2 / (u3);
    % C = (a*A - b*B) / ( (a^2) + (b^2)) ;
    % 
    % roll = atan( (B + b*C) / a );
    % pitch = atan( C * cos(roll) );

    roll = asin( (u2*m) / ft );
    pitch = asin( (-u1*m) / (ft*cos(roll)) );
    r_yaw = 0;

    % Smoothing Factor ( Use exponential decay, just to start from zero )
    % roll = roll * (1-exp(-Ts));
    % pitch = pitch * (1-exp(-Ts));
    % r_yaw = r_yaw * (1-exp(-Ts));

    % Saturation
    if roll > pi/10
        roll = pi/10;
    elseif roll < -pi/10
        roll = -pi/10;
    end

    if pitch > pi/10
        pitch = pi/10;
    elseif pitch < -pi/10
        pitch = -pi/10;
    end

end

% function [ft, pitch, roll] = system_solve(u1, u2, u3, psi, m) % u1 = ux , u2 = uy , u3 = uz - g  
%     if psi <= 0.001 && psi >= -0.001
%         psi = 0.001;
%     end
%     a = sin(psi);
%     b = cos(psi);
% 
%     A = u1 / (u3);
%     B = u2 / (u3);
%     C = (a*A - b*B) / ( (a^2) + (b^2)) ;
% 
%     roll = atan( (B + b*C) / a );
%     pitch = atan( C * cos(roll) );
% 
%     % saftey limit threshold on desired pitch and roll
%     if pitch>pi/4
%         pitch = pi/4;
%     elseif pitch<-pi/4
%         pitch = -pi/4;
%     end
%     if roll>pi/4
%         roll = pi/4;
%     elseif roll<-pi/4
%         roll = -pi/4;
%     end
%     ft = ( m / (cos(pitch)*cos(roll)) ) * (-u3); 
% end

== matlab function Sim_PA_DDPG_4drone/leader 1/Drone Dynamics/MATLAB Function3 ==
  settings: updateMethod=DISCRETE
  data: state_vector input; noisy_vector output; noise_percent input
function noisy_vector = add_state_noise(state_vector,noise_percent)

    sensor_uncert = [0.02, 0.02, 0.05, 0.05, 0.05, 0.05, 0.15, 0.15, 0.5, 0.005, 0.005, 0.005]';
  
    noise = (noise_percent) * sensor_uncert .* randn(size(state_vector)); % 0.01 usually add noise_percent 1 2 3 4 5
    noisy_vector = state_vector + noise;

end

== matlab function Sim_PA_DDPG_4drone/Reference1/Position Reference Signal ==
  data: t input; x_desired output; y_desired output; z_desired output; xdot_desired output; ydot_desired output; zdot_desired output
function [x_desired, y_desired, z_desired, xdot_desired, ydot_desired, zdot_desired] = trajectory_generator(t)

    % x_desired    = 9.81 * (1-exp(-0.01*t)) * cos(0.2*t);
    % xdot_desired = 9.81 * ( (0.01*exp(-0.01*t)*cos(0.2*t)) - (0.2*(1-exp(-0.01*t))*sin(0.2*t)) );
    % 
    % y_desired    = 9.81 * (1-exp(-0.01*t)) * sin(0.2*t);
    % ydot_desired = 9.81 * ( (0.01*exp(-0.01*t)*sin(0.2*t)) + (0.2*(1-exp(-0.01*t))*cos(0.2*t)) );
    % 
    % z_desired    = -1*t;
    % zdot_desired = -1;

        %% crown path 
    x_desired = 9.81*cos(0.2*t);
    xdot_desired = -1.962*sin(0.2*t);

    y_desired = 9.81*sin(0.2*t);
    ydot_desired =  1.962*cos(0.2*t);
    
    z_desired = -4*cos(1*t)-9.81;
    zdot_desired = 4*sin(t);

end


% ref = @(t) [(1-exp(-0.01*t))*9.81*cos(0.2*t);
%             (1-exp(-0.01*t))*9.81*sin(0.2*t);
%             -.1*t];


 % x_desired    = 9.81 * (1-exp(-0.01*t)) * cos(0.2*t);
 %    xdot_desired = 9.81 * ( (0.01*exp(-0.01*t)*cos(0.2*t)) - (0.2*(1-exp(-0.01*t))*sin(0.2*t)) );
 % 
 %    y_desired    = 9.81 * (1-exp(-0.01*t)) * sin(0.2*t);
 %    ydot_desired = 9.81 * ( (0.01*exp(-0.01*t)*sin(0.2*t)) + (0.2*(1-exp(-0.01*t))*cos(0.2*t)) );
 % 
 %    z_desired    = -0.1*t;
 %    zdot_desired = -0.1;

== matlab function Sim_PA_DDPG_4drone/leader 1/Drone Dynamics/MATLAB Function4 ==
  settings: updateMethod=DISCRETE
  data: control_vector input; noisy_vector output; noise_percent input
function noisy_vector = add_control_noise(control_vector, noise_percent)

    L = 0.2;
    % drag = 0.02; % (drag coef)
    max_Ft = 2*9.81;
    Tmax = max_Ft/4;
    Max_torque = Tmax*L*2;
    actuator_uncert = [0.1*max_Ft, 0.01*Max_torque, 0.01*Max_torque, 0.02*Max_torque]';
    
    noise = (noise_percent) * actuator_uncert .* randn(size(control_vector)); % noise_percent 1 2 3 4 5
    noisy_vector = control_vector + noise;
    
end

== matlab function Sim_PA_DDPG_4drone/leader 1/Drone Dynamics/MATLAB Function5 ==
  data: X input; Wxyz input; X output; Ts_Sim input; wind_logic input
function X = wind_f_m( X,Wxyz, Ts_Sim,  wind_logic)

    Cd = [.8; 0.8;1.2]; % Drag coefficient
    L = 0.2; % Half arm length (m)
    h = 0.05;
    A = [L*2*h, L*2*h, 2*L*L]; % Approximate frontal areas [x, y, z] in m^2
    r = [ L,  L, -L, -L;   % X positions of motors
          L, -L, -L,  L;   % Y positions of motors
          0,  0,  0,  0 ]; % Z positions (motors at same height)
    rho = 1.225; % Air density (kg/m^3)

    Ix = 0.3; Iy = 0.4; Iz = 0.5; m = 1;
    if wind_logic ==1
        R = eul2rotm_zyx( X(7), X(8), X(9) );
        Wxyz_body = R'*Wxyz;
        V_rel = X(4:6) - Wxyz_body;
        F_wind = -0.5 * rho * Cd .*diag(A) * (V_rel .* abs(V_rel)); % Compute wind forces
        
        F_wind_motors = repmat(F_wind, 1, 4) + 0.01*randn(3,4);
    
        M_wind_motors = cross(r, F_wind_motors, 1);
        M_wind = sum(M_wind_motors, 2);  
        
        accn_dist = F_wind/m;
        alpha_dist=    [M_wind(1)/Ix;
                        M_wind(2)/Iy;
                        M_wind(3)/Iz];
    
        X = X + Ts_Sim * [0;0;0;
                         accn_dist;
                         0;0;0;
                         alpha_dist];
    end
end

== matlab function Sim_PA_DDPG_4drone/leader 1/Drone Dynamics/MATLAB Function6 ==
  data: U input; out output; logic input
% saturation function
function out = saturate_controls(U, logic)

    if logic == 1

        ft = U(1);
        torques = [U(2); U(3); U(4)];
        m = 1;
        g = 9.81;
        L = 0.2;
        drag = 0.02; % (drag coef)
        max_Ft = 2*m*g;
        Tmin = 0;
        Tmax = max_Ft/4;
        max_torque = Tmax*L*2;
        max_yaw_torque = 0.7*max_torque;

        % saturate the torques to the max torque the drone can produce
        for p = 1:2 % sat the first 2
            if torques(p) > max_torque
                torques(p) = max_torque;
            elseif torques(p) < -max_torque
                torques(p) = -max_torque;
            end
        end
        if torques(3) > max_yaw_torque
            torques(3) = max_yaw_torque;
        elseif torques(3) < -max_yaw_torque
            torques(3) = -max_yaw_torque;
        end
        % solve for the thrust of each motor given those torques
        T1 = (ft - torques(1)/(2*L) - torques(2)/(2*L) + torques(3)/(4*drag)) / 4;
        T2 = (ft - torques(1)/(2*L) + torques(2)/(2*L) + torques(3)/(4*drag)) / 4;
        T3 = (ft + torques(1)/(2*L) - torques(2)/(2*L) - torques(3)/(4*drag)) / 4;
        T4 = (ft + torques(1)/(2*L) + torques(2)/(2*L) - torques(3)/(4*drag)) / 4;
        each_motor_thrust = [T1;T2;T3;T4];

        % saturate each motor thrust to its bounded values
        for j = 1:4
            if each_motor_thrust(j) > Tmax
                each_motor_thrust(j) = Tmax;
            elseif each_motor_thrust(j) < Tmin
                each_motor_thrust(j) = Tmin;
            end
        end

        ft = sum(each_motor_thrust);

        if ft>max_Ft
            ft = max_Ft;
        elseif ft<0
            ft = 0;
        end

        out = [ft; torques];

    else
    
        out = U;
    
    end


end
